simulink model "Foc_model_Matlab_3"  (R2024b)
settings: Solver=FixedStepDiscrete  StartTime=0.0  StopTime=5  FixedStep=Ts_simulink  RelTol=1e-3  EnableMultiTasking=on
PreLoadFcn:
  | mcb_pmsm_foc_hall_S32K144EVB_data;
InitFcn:
  | mbd_s32k_consistency_checks(bdroot(gcs));
model workspace (MAT data in the model file):
  IDC_OVERCURRENT : Simulink.Parameter (value not decoded)
  VDC_OVERVOLTAGE : Simulink.Parameter (value not decoded)
  VDC_UNDERVOLTAGE : Simulink.Parameter (value not decoded)
undefined symbols (not defined in the file or in its folder): Aw, Bw, DiscIntNeverNeededParam, External, inverter, Kcd, Kcq, Kcs, Kid, Kiq, LQFP, mcb_isCodeGenVar, mcb_isSimVar, One, PI_params, pmsm, PU_System, rhow, Shot, sigbuilder_block, TRGMUX_PDB_TRIG, Ts, Ts_motor, Ts_simulink, Ts_speed, tuning
libraries: mbd_s32k1xx_ec_toolbox x39, mcbcontrolslib x9, simulink x6, mcbpositiondecoderlib x6, mbd_msd_ec_toolbox x5, hdlsllib x4, slpidlib x2, mcbhdlpositiondecoderlib x1, mcbplantlib x1, autolibpmsmexterior x1
(part 2 of 3)

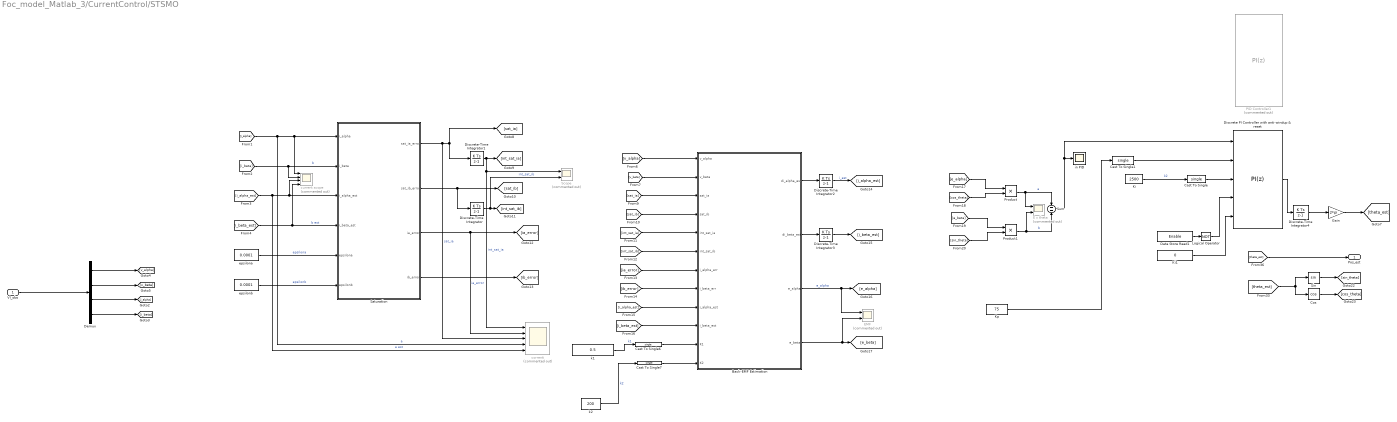
== system Foc_model_Matlab_3/CurrentControl/STSMO ==
  VI_obs : Inport
  Back-EMF Estimation : MATLAB Function  TreatAsAtomicUnit=on
  Cast To Single{,1,6..7} (4 alike) : DataTypeConversion  OutDataTypeStr=single  SaturateOnIntegerOverflow=off  RndMeth=Floor
  Cos : Trigonometry  Operator=cos
  Data Store Read1 : DataStoreRead  DataStoreName=Enable  IndexOptions=Index vector (dialog)  Indices=1  OutputSizes=1
  Demux : Demux
  Discrete PI Controller with anti-windup & reset : slpidlib/PID Controller  Controller=PI  Form=Parallel  TimeDomain=Discrete-time  UseExternalTs=off  SampleTime=-1  IntegratorMethod=Forward Euler  FilterMethod=Forward Euler  ControllerParametersSource=external  P=1  I=1  UseKiTs=off  D=0  UseExternalDerivativeSource=off  N=100  UseFilter=on  TunerSelectOption=Transfer Function Based (PID Tuner App)  InitialConditionSource=external  InitialConditionForIntegrator=0  InitialConditionForFilter=0  DifferentiatorICPrevScaledInput=0  ExternalReset=level  TrackingMode=off  Kt=1  LimitOutput=off  SatLimitsSource=internal  UpperSaturationLimit=1  LowerSaturationLimit=-1  LinearizeAsGain=on  AntiWindupMode=clamping  Kb=1  LimitIntegrator=off  UpperIntegratorSaturationLimit=inf  LowerIntegratorSaturationLimit=-inf  RndMeth=Simplest  POutMin=[]  POutMax=[]  IOutMin=[]  IOutMax=[]  DOutMin=[]  DOutMax=[]  NOutMin=[]  NOutMax=[]  SumOutMin=[]  SumOutMax=[]  SaturationOutDataTypeStr=Inherit: Inherit via back propagation  SaturationOutMin=[]  SaturationOutMax=[]  PParamMin=[]  PParamMax=[]  IParamMin=[]  IParamMax=[]  DParamMin=[]  DParamMax=[]  NParamMin=[]  NParamMax=[]  KbParamMin=[]  KbParamMax=[]  KtParamMin=[]  KtParamMax=[]  KbOutMin=[]  KbOutMax=[]  KtOutMin=[]  KtOutMax=[]  IntegratorOutMin=[]  IntegratorOutMax=[]  FilterOutMin=[]  FilterOutMax=[]  SumI1OutMin=[]  SumI1OutMax=[]  SumI2OutMin=[]  SumI2OutMax=[]  SumI3OutMin=[]  SumI3OutMax=[]  SumI4OutMin=[]  SumI4OutMax=[]  SumDOutMin=[]  SumDOutMax=[]  DifferentiatorOutMin=[]  DifferentiatorOutMax=[]  FilterDiffOutCoefMin=[]  FilterDiffOutCoefMax=[]  ReciprocalOutMin=[]  ReciprocalOutMax=[]  SumDenOutMin=[]  SumDenOutMax=[]  SumNumOutMin=[]  SumNumOutMax=[]  DivideOutMin=[]  DivideOutMax=[]  UdiffTsProdOutMin=[]  UdiffTsProdOutMax=[]  NTsProdOutMin=[]  NTsProdOutMax=[]  UintegralTsProdOutMin=[]  UintegralTsProdOutMax=[]  UngainTsProdOutMin=[]  UngainTsProdOutMax=[]  ClampingZeroOutDataTypeStr=Inherit: Inherit via back propagation  ClampingZeroOutMin=[]  ClampingZeroOutMax=[]  FilterDenConstantOutDataTypeStr=Inherit: Inherit via back propagation  FilterDenConstantOutMin=[]  FilterDenConstantOutMax=[]  PCopyOutDataTypeStr=Inherit: Inherit via back propagation  PCopyOutMin=[]  PCopyOutMax=[]  NCopyOutDataTypeStr=Inherit: Inherit via back propagation  NCopyOutMin=[]  NCopyOutMax=[]  IntegratorContinuousStateAttributes=''  IntegratorStateMustResolveToSignalObject=off  IntegratorRTWStateStorageClass=Auto  FilterContinuousStateAttributes=''  FilterStateMustResolveToSignalObject=off  FilterRTWStateStorageClass=Auto  ParallelPVariant=ExternalParameters  IdealPVariant=Disabled  IVariant=ExternalParameters  DVariant=Disabled  IntegratorVariant=Discrete  SatVariant=Disabled  AWVariant=Passthrough  PCopyVariant=Disabled  TRVariant=Disabled  FdbkBlocksVariant=Forward  IdealPFdbkVariant=Disabled  SatFdbkVariant=Disabled  DerivativeFilterVariant=Disabled  NVariant=Disabled  NCopyVariant=Disabled_SignalSpec  FilterICVariant=Disabled  IntegratorICVariant=ExternalICs  ExternalResetVariant=ExternalReset  TRSumVariant=Passthrough  SumFdbkVariant=Disabled  SumVariant=Sum_PI  TsampFilterVariant=InternalTs  TsampNgainVariant=Passthrough  TsampIntegralVariant=Disabled_SignalSpec  ExternalSaturationOutDataTypeStr=Inherit: Same as second input  DerivativeSourceVariant=Disabled  PreIntVariant=InternalPreInt
  Discrete-Time Integrator{,1..4} (5 alike) : DiscreteIntegrator  SampleTime=-1  ICPrevOutput=DiscIntNeverNeededParam  ICPrevScaledInput=DiscIntNeverNeededParam
  E x theta : Scope  Commented=on  NumInputPorts=2
  EMF : Scope  Commented=on  NumInputPorts=2
  Gain : Gain  Gain=2*pi
  Ki : Constant  Value=2500
  Ki1 : Constant  Value=0  OutDataTypeStr=dataType  SampleTime=-1
  Kp : Constant  Value=75
  Logical Operator : Logic  Operator=NOT  IconShape=distinctive  AllPortsSameDT=off  OutDataTypeStr=boolean
  PID Controller1 : slpidlib/PID Controller  Commented=on  Controller=PI  Form=Parallel  TimeDomain=Discrete-time  UseExternalTs=off  SampleTime=-1  IntegratorMethod=Forward Euler  FilterMethod=Forward Euler  ControllerParametersSource=external  P=1  I=1  UseKiTs=off  D=0  UseExternalDerivativeSource=off  N=100  UseFilter=on  TunerSelectOption=Transfer Function Based (PID Tuner App)  InitialConditionSource=internal  InitialConditionForIntegrator=0  InitialConditionForFilter=0  DifferentiatorICPrevScaledInput=0  ExternalReset=none  TrackingMode=off  Kt=1  LimitOutput=off  SatLimitsSource=internal  UpperSaturationLimit=inf  LowerSaturationLimit=-inf  LinearizeAsGain=on  AntiWindupMode=none  Kb=1  LimitIntegrator=off  UpperIntegratorSaturationLimit=inf  LowerIntegratorSaturationLimit=-inf  POutMin=[]  POutMax=[]  IOutMin=[]  IOutMax=[]  DOutMin=[]  DOutMax=[]  NOutMin=[]  NOutMax=[]  SumOutMin=[]  SumOutMax=[]  SaturationOutMin=[]  SaturationOutMax=[]  PParamMin=[]  PParamMax=[]  IParamMin=[]  IParamMax=[]  DParamMin=[]  DParamMax=[]  NParamMin=[]  NParamMax=[]  KbParamMin=[]  KbParamMax=[]  KtParamMin=[]  KtParamMax=[]  KbOutMin=[]  KbOutMax=[]  KtOutMin=[]  KtOutMax=[]  IntegratorOutMin=[]  IntegratorOutMax=[]  FilterOutMin=[]  FilterOutMax=[]  SumI1OutMin=[]  SumI1OutMax=[]  SumI2OutMin=[]  SumI2OutMax=[]  SumI3OutMin=[]  SumI3OutMax=[]  SumI4OutMin=[]  SumI4OutMax=[]  SumDOutMin=[]  SumDOutMax=[]  DifferentiatorOutMin=[]  DifferentiatorOutMax=[]  FilterDiffOutCoefMin=[]  FilterDiffOutCoefMax=[]  ReciprocalOutMin=[]  ReciprocalOutMax=[]  SumDenOutMin=[]  SumDenOutMax=[]  SumNumOutMin=[]  SumNumOutMax=[]  DivideOutMin=[]  DivideOutMax=[]  UdiffTsProdOutMin=[]  UdiffTsProdOutMax=[]  NTsProdOutMin=[]  NTsProdOutMax=[]  UintegralTsProdOutMin=[]  UintegralTsProdOutMax=[]  UngainTsProdOutMin=[]  UngainTsProdOutMax=[]  ClampingZeroOutDataTypeStr=Inherit: Inherit via back propagation  ClampingZeroOutMin=[]  ClampingZeroOutMax=[]  FilterDenConstantOutDataTypeStr=Inherit: Inherit via back propagation  FilterDenConstantOutMin=[]  FilterDenConstantOutMax=[]  PCopyOutDataTypeStr=Inherit: Inherit via back propagation  PCopyOutMin=[]  PCopyOutMax=[]  NCopyOutDataTypeStr=Inherit: Inherit via back propagation  NCopyOutMin=[]  NCopyOutMax=[]  IntegratorContinuousStateAttributes=''  IntegratorStateMustResolveToSignalObject=off  IntegratorRTWStateStorageClass=Auto  FilterContinuousStateAttributes=''  FilterStateMustResolveToSignalObject=off  FilterRTWStateStorageClass=Auto  ParallelPVariant=ExternalParameters  IdealPVariant=Disabled  IVariant=ExternalParameters  DVariant=Disabled  IntegratorVariant=Discrete  SatVariant=Disabled  AWVariant=Passthrough  PCopyVariant=Disabled  TRVariant=Disabled  FdbkBlocksVariant=Forward  IdealPFdbkVariant=Disabled  SatFdbkVariant=Disabled  DerivativeFilterVariant=Disabled  NVariant=Disabled  NCopyVariant=Disabled_SignalSpec  FilterICVariant=Disabled  IntegratorICVariant=InternalICs  ExternalResetVariant=Disabled  TRSumVariant=Passthrough  SumFdbkVariant=Disabled  SumVariant=Sum_PI  TsampFilterVariant=InternalTs  TsampNgainVariant=Passthrough  TsampIntegralVariant=Disabled_SignalSpec  ExternalSaturationOutDataTypeStr=Inherit: Same as second input  DerivativeSourceVariant=Disabled  PreIntVariant=InternalPreInt
  Product : Product
  Product1 : Product
  "Saturation " : MATLAB Function  TreatAsAtomicUnit=on
  Scope : Scope  Commented=on  NumInputPorts=2
  Sin : Trigonometry
  Sum : Sum  Inputs=--
  correnti : Scope  Commented=on  NumInputPorts=5
  current scope : Scope  Commented=on  NumInputPorts=4
  epsilona : Constant  Value=0.0001
  epsilonb : Constant  Value=0.0001
  in PID : Scope
  k1 : Constant  Value=0.5
  k2 : Constant  Value=200
  Pos_est : Outport
  wires:
  Demux/4 -> [i_beta]
  [i_beta] -> current scope/2, "Saturation "/2(i_beta)  "b"
  "Saturation "/1(sat_ia_error) -> correnti/3, Discrete-Time Integrator1/1, [sat_ia]  "sat_ia"
  "Saturation "/2(sat_ib_error) -> Discrete-Time Integrator/1, [sat_ib]
  "Saturation "/3(ia_error) -> correnti/2, [ia_error]  "ia_error"
  "Saturation "/4(ib_error) -> [ib_error]
  Discrete-Time Integrator/1 -> Scope/2, [int_sat_ib]  "int_sat_ib"
  Back-EMF Estimation/1(di_alpha_est) -> Discrete-Time Integrator2/1
  Back-EMF Estimation/2(di_beta_est) -> Discrete-Time Integrator3/1
  Back-EMF Estimation/3(e_alpha) -> EMF/1, [e_alpha]  "e_alpha"
  Back-EMF Estimation/4(e_beta) -> EMF/2, [e_beta]
  [v_alpha] -> Back-EMF Estimation/1(v_alpha)
  [v_beta] -> Back-EMF Estimation/2(v_beta)
  [sat_ia] -> Back-EMF Estimation/3(sat_ia)
  [sat_ib] -> Back-EMF Estimation/4(sat_ib)
  [int_sat_ia] -> Back-EMF Estimation/5(int_sat_ia)
  [int_sat_ib] -> Back-EMF Estimation/6(int_sat_ib)
  [ia_error] -> Back-EMF Estimation/7(i_alpha_err)
  [ib_error] -> Back-EMF Estimation/8(i_beta_err)
  [sin_theta] -> Product1/2
  [cos_theta] -> Product/2
  VI_obs/1 -> Demux/1
  Sin/1 -> [sin_theta]
  Cos/1 -> [cos_theta]
  [theta_est] -> Pos_est/1
  k1/1 -> Cast To Single6/1  "k1"
  k2/1 -> Cast To Single7/1  "k2"
  epsilona/1 -> "Saturation "/5(epsilona)  "epsilona"
  epsilonb/1 -> "Saturation "/6(epsilonb)  "epsilonb"
  Demux/2 -> [v_beta]
  Demux/1 -> [v_alpha]
  Cast To Single6/1 -> Back-EMF Estimation/11(K1)
  Cast To Single7/1 -> Back-EMF Estimation/12(K2)
  Demux/3 -> [i_alpha]
  [i_alpha_est] -> Back-EMF Estimation/9(i_alpha_est)
  [i_beta_est] -> Back-EMF Estimation/10(i_beta_est)
  Product1/1 -> E x theta/2, Sum/2  "b"
  Discrete-Time Integrator3/1 -> [i_beta_est]
  Discrete-Time Integrator2/1 -> [i_alpha_est]  "i_est"
  [e_beta] -> Product1/1
  [e_alpha] -> Product/1
  [i_beta_est] -> current scope/4, "Saturation "/4(i_beta_est)  "b est"
  [i_alpha_est] -> correnti/5, current scope/3, "Saturation "/3(i_alpha_est)  "a est"
  Kp/1 -> Cast To Single1/1
  [i_alpha] -> correnti/4, current scope/1, "Saturation "/1(i_alpha)  "a"
  Discrete-Time Integrator1/1 -> correnti/1, Scope/1, [int_sat_ia]  "int_sat_ia"
  [theta_est] -> Sin/1, Cos/1
  Product/1 -> E x theta/1, Sum/1  "a"
  Cast To Single1/1 -> Discrete PI Controller with anti-windup & reset/2
  Sum/1 -> Discrete PI Controller with anti-windup & reset/1, in PID/1
  Cast To Single/1 -> Discrete PI Controller with anti-windup & reset/3
  Discrete PI Controller with anti-windup & reset/1 -> Discrete-Time Integrator4/1
  Discrete-Time Integrator4/1 -> Gain/1
  Gain/1 -> [theta_est]
  Ki/1 -> Cast To Single/1  "k2"
  Logical Operator/1 -> Discrete PI Controller with anti-windup & reset/4
  Ki1/1 -> Discrete PI Controller with anti-windup & reset/5
  Data Store Read1/1 -> Logical Operator/1

== system Foc_model_Matlab_3/CurrentControl/Sensor Driver Blocks ==
  Sensor Driver Blocks (codegen) : Subsystem  VariantControl=mcb_isCodeGenVar()
  Sensor Driver Blocks (sim) : Subsystem  VariantControl=mcb_isSimVar()
  Iab_Meas_ADC : Outport

== system Foc_model_Matlab_3/Hall Sensor/CodeGen ==
  Add1 : Sum  Inputs=+++  OutDataTypeStr=Inherit: Inherit via back propagation
  Bit Shift : hdlsllib/Logic and Bit Operations/Bit Shift  mode=Shift Left Logical  N=2
  Bit Shift1 : hdlsllib/Logic and Bit Operations/Bit Shift  mode=Shift Left Logical  N=1
  Data Type Conversion2 : DataTypeConversion  OutDataTypeStr=uint32  SaturateOnIntegerOverflow=off  RndMeth=Floor
  Data Type Conversion3 : DataTypeConversion  OutDataTypeStr=uint32  SaturateOnIntegerOverflow=off  RndMeth=Floor
  Data Type Conversion6 : DataTypeConversion  OutDataTypeStr=uint32  SaturateOnIntegerOverflow=off  RndMeth=Floor
  Digital_Input_HALL_A : mbd_s32k1xx_ec_toolbox/GPIO Blocks/Digital_Input  gpio_pin=PTA1: [PTA1 | Port A I/O]  pull_resistor=None  passive_filter=off
  Digital_Input_HALL_B : mbd_s32k1xx_ec_toolbox/GPIO Blocks/Digital_Input  gpio_pin=PTD10: [PTD10 | Port D I/O]  pull_resistor=None  passive_filter=off
  Digital_Input_HALL_C : mbd_s32k1xx_ec_toolbox/GPIO Blocks/Digital_Input  gpio_pin=PTD11: [PTD11 | Port D I/O]  pull_resistor=None  passive_filter=off
  Out1 : Outport
  wires:
  Bit Shift1/1 -> Add1/2  "HALL_B"
  Digital_Input_HALL_B/1 -> Data Type Conversion2/1
  Add1/1 -> Out1/1
  Data Type Conversion6/1 -> Add1/3  "HALL_C"
  Digital_Input_HALL_A/1 -> Data Type Conversion3/1
  Data Type Conversion2/1 -> Bit Shift1/1
  Bit Shift/1 -> Add1/1  "HALL_A"
  Digital_Input_HALL_C/1 -> Data Type Conversion6/1
  Data Type Conversion3/1 -> Bit Shift/1

== system Foc_model_Matlab_3/Hall Sensor/Sim ==
  Data Type Conversion1 : DataTypeConversion  OutDataTypeStr=uint32  SaturateOnIntegerOverflow=off  RndMeth=Floor
  Ground : Ground
  Out1 : Outport
  wires:
  Ground/1 -> Data Type Conversion1/1
  Data Type Conversion1/1 -> Out1/1

== system Foc_model_Matlab_3/HallCodeGen/Subsystem2 ==
  ADC1_IRQHandler : Subsystem  TreatAsAtomicUnit=on
  ADC1_ISR : mbd_s32k1xx_ec_toolbox/Motor Control Blocks/ADC Blocks/ADC_ISR  instance=1  pri=5  sc1n=C
  Data Store Write : DataStoreWrite  DataStoreName=ADC_A  IndexOptions=Index vector (dialog)  Indices=1  OutputSizes=1
  Data Store Write1 : DataStoreWrite  DataStoreName=ADC_B  IndexOptions=Index vector (dialog)  Indices=1  OutputSizes=1
  Data Type Conversion : DataTypeConversion  OutDataTypeStr=single  SaturateOnIntegerOverflow=off  RndMeth=Floor
  Demux : Demux  Outputs=2
  PDB1_IRQHandler : Subsystem  TreatAsAtomicUnit=on
  PDB1_ISR : mbd_s32k1xx_ec_toolbox/Motor Control Blocks/PDB Blocks/PDB_ISR  Priority=8  pdbModule=0  prioInterrupt=6  regScPdbie=on  regScPdbeie=off  regIdlyIdly=4999
  Terminator{,1..2,6} (4 alike) : Terminator
  FcnCall : Outport  VectorParamsAs1DForOutWhenUnconnected=off
  wires:
  ADC1_IRQHandler/2(ADC_res) -> Data Type Conversion/1
  PDB1_ISR/1 -> PDB1_IRQHandler/Trigger
  PDB1_ISR/3 -> Terminator2/1  "CH0S_ERR"
  PDB1_ISR/4 -> Terminator/1  "CH1S_ERR"
  ADC1_ISR/1 -> ADC1_IRQHandler/Trigger
  PDB1_ISR/2 -> Terminator1/1  "SC_PDBIF"
  ADC1_ISR/2 -> ADC1_IRQHandler/1(ADC_IB)
  ADC1_IRQHandler/1(ADC_Event) -> FcnCall/1
  ADC1_ISR/3 -> Terminator6/1
  Demux/2 -> Data Store Write1/1
  Data Type Conversion/1 -> Demux/1
  Demux/1 -> Data Store Write/1

== system Foc_model_Matlab_3/Hardware Initialization/FAULT ==
  Action Port : ActionPort  ActionPortLabel=else
  LED_GREEN : mbd_s32k1xx_ec_toolbox/GPIO Blocks/Digital_Output  gpio_pin=PTD16: [PTD16 | Port D I/O]  init_val=Low  drive_strength=Low
  LED_RED : mbd_s32k1xx_ec_toolbox/GPIO Blocks/Digital_Output  gpio_pin=PTD15: [PTD15 | Port D I/O]  init_val=Low  drive_strength=Low
  OFF : Constant  OutDataTypeStr=boolean
  ON : Constant  Value=0  OutDataTypeStr=boolean
  wires:
  OFF/1 -> LED_GREEN/1
  ON/1 -> LED_RED/1

== system Foc_model_Matlab_3/Hardware Initialization/GD3000_interrupt ==
  function : TriggerPort  TriggerType=function-call  VariantControl=Variant
  FAULT_write : DataStoreWrite  DataStoreName=FAULT  IndexOptions=Index vector (dialog)  Indices=1  OutputSizes=1
  FTM_PWM_Disable_Enable : mbd_s32k1xx_ec_toolbox/Motor Control Blocks/FTM Blocks/FTM_PWM_Disable_Enable  ftmModule=3  action=Disable
  NOK : Constant  OutDataTypeStr=boolean
  TPP_Functional_Mode : mbd_msd_ec_toolbox/TPP/TPP_Functional_Mode  tppInstance=0  action=Sleep
  wires:
  NOK/1 -> FAULT_write/1

== system Foc_model_Matlab_3/Hardware Initialization/If Action Subsystem ==
  Action Port : ActionPort  ActionPortLabel=if(u1 == 0)
  LED_GREEN : Constant  Value=0  OutDataTypeStr=boolean  SampleTime=-1
  LED_GREEN_ON : mbd_s32k1xx_ec_toolbox/GPIO Blocks/Digital_Output  gpio_pin=PTD16: [PTD16 | Port D I/O]  init_val=Low  drive_strength=Low
  LED_RED : Constant  OutDataTypeStr=boolean  SampleTime=-1
  LED_RED_OFF : mbd_s32k1xx_ec_toolbox/GPIO Blocks/Digital_Output  gpio_pin=PTD15: [PTD15 | Port D I/O]  init_val=Low  drive_strength=Low
  wires:
  LED_GREEN/1 -> LED_GREEN_ON/1
  LED_RED/1 -> LED_RED_OFF/1

== system Foc_model_Matlab_3/Hardware Initialization/enable_FTM_PDB_ADC_triggering ==
  function : TriggerPort  TriggerType=function-call  VariantControl=(inherit)
  Custom code to reload the PDB value : Subsystem  Priority=6  mask(System Outputs){ShowInLibBrowser=0}
      mask prompts: ShowInLibBrowser "Simulink:masks:CustCodeMaskParam1_MP"
      settings: CopyFcn=cccopyfcn(gcb)  OpenFcn=ccopenfcn('System Outputs Function')
      mask Help: eval('feval(''rtwprivate'',''rtwhelpview'',''rtw_sys_outputs_block'')');
      mask Display: disp('System\nOutputs');
  FTM_Init_Trigger_Disable_Enable : mbd_s32k1xx_ec_toolbox/Motor Control Blocks/FTM Blocks/FTM_Init_Trigger_Disable_Enable  Priority=3  ftmModule=3  action=Enable
  FTM_PWM_Disable_Enable : mbd_s32k1xx_ec_toolbox/Motor Control Blocks/FTM Blocks/FTM_PWM_Disable_Enable  Priority=1  ftmModule=3  action=Enable
  PDB0_Enable : mbd_s32k1xx_ec_toolbox/Motor Control Blocks/PDB Blocks/PDB_Enable  Priority=4  pdbModule=0  pdbAction=Enable
  PDB1_Enable : mbd_s32k1xx_ec_toolbox/Motor Control Blocks/PDB Blocks/PDB_Enable  Priority=5  pdbModule=1  pdbAction=Enable
  TPP_ISR_Enable_Disable : mbd_msd_ec_toolbox/TPP/TPP_ISR_Enable_Disable  Priority=7  tppInstance=0  mcuTppIntEn=on  prioInt=15

== system Foc_model_Matlab_3/Inverter and Motor - Plant Model/Codegeneration ==
  Duty_Cycles : Inport
  Ground : Ground
  Ground1 : Ground
  Terminator : Terminator
  Iab_fb_Sim : Outport  VectorParamsAs1DForOutWhenUnconnected=off
  Pos_fb_Sim : Outport  Port=2  VectorParamsAs1DForOutWhenUnconnected=off
  wires:
  Duty_Cycles/1 -> Terminator/1
  Ground/1 -> Iab_fb_Sim/1
  Ground1/1 -> Pos_fb_Sim/1

== system Foc_model_Matlab_3/Inverter and Motor - Plant Model/Simulation ==
  Duty_Cycles : Inport
  Average Inverter : Subsystem
  Load_Profile (Torque) : Subsystem
  RT1 : RateTransition  Deterministic=off  OutPortSampleTime=Ts_simulink
  RT3 : RateTransition  Deterministic=off  OutPortSampleTime=Ts_simulink
  Rate Transition : RateTransition  Deterministic=off  OutPortSampleTime=Ts_motor
  Rate Transition1 : RateTransition  Deterministic=off  OutPortSampleTime=Ts_motor
  Sensor_Measurements : Subsystem
  Surface Mount PMSM : autolibpmsmexterior/Surface Mount PMSM  port_config=Torque  sim_type=Discrete  Ts=Ts_motor  FilePath=surfacepmsm_motordata.m  P=pmsm.p  Rs=pmsm.Rs + inverter.R_board  Ldq_=pmsm.Ld  KConstText=Permanent flux linkage constant (lambda_pm):  lambda_pm=pmsm.FluxPM  Ke=159.9771  Kt=1.323  mechanical=[pmsm.J, pmsm.B, 0]  idq0=[0 0]  theta_init=0  omega_init=0  KConst=pmsm.FluxPM  lambda_pm_calc=pmsm.FluxPM  RefBlkName='autolibpmsmexterior/Surface Mount PMSM'  aMode=5  Ldq="[0.0006      0.0006]"
  Terminator : Terminator
  Iab_fb_Sim : Outport  VectorParamsAs1DForOutWhenUnconnected=off
  Pos_fb_Sim : Outport  Port=2  VectorParamsAs1DForOutWhenUnconnected=off
  wires:
  RT1/1 -> Sensor_Measurements/2(PhaseCurr)
  Surface Mount PMSM/3 -> Terminator/1
  Average Inverter/1(Vabc) -> Rate Transition/1
  Load_Profile (Torque)/1(Load_Trq) -> Rate Transition1/1
  Surface Mount PMSM/2 -> RT1/1  "Iabc"
  RT3/1 -> Sensor_Measurements/1(Info)
  Surface Mount PMSM/1 -> RT3/1
  Rate Transition1/1 -> Surface Mount PMSM/1
  Rate Transition/1 -> Surface Mount PMSM/2
  Duty_Cycles/1 -> Average Inverter/1(Duty_abc)
  Sensor_Measurements/1(Iab_fb) -> Iab_fb_Sim/1
  Sensor_Measurements/2(Pos_fb) -> Pos_fb_Sim/1

== system Foc_model_Matlab_3/Serial Receive/Code Generation ==
  Data Store Read2 : DataStoreRead  DataStoreName=DesiredSpeed  IndexOptions=Index vector (dialog)  Indices=1  OutputSizes=1
  Data Store Read3 : DataStoreRead  DataStoreName=Enable  IndexOptions=Index vector (dialog)  Indices=1  OutputSizes=1
  Data Type Conversion5 : DataTypeConversion  OutDataTypeStr=single  RndMeth=Simplest  SaturateOnIntegerOverflow=off
  Mux1 : Mux  Inputs=2
  rpm2PU : Gain  Gain=1/pmsm.N_max  RndMeth=Simplest
  Data : Outport
  wires:
  Data Store Read3/1 -> Data Type Conversion5/1
  Data Type Conversion5/1 -> Mux1/2
  Mux1/1 -> Data/1
  Data Store Read2/1 -> rpm2PU/1
  rpm2PU/1 -> Mux1/1

== system Foc_model_Matlab_3/Serial Receive/Simulation ==
  Cast To Single1 : DataTypeConversion  OutDataTypeStr=single  SaturateOnIntegerOverflow=off  RndMeth=Floor
  Constant : Constant
  Gain : Gain  Gain=1/pmsm.N_max
  Mux2 : Mux  Inputs=2
  Push Button : PushButtonBlock  ButtonType=Latch  OffValue=0.000000
  Signal Builder : Subsystem  Tag=STV Subsys  LoadFcn=sigbuilder_block('load');  StartFcn=sigbuilder_block('start');  StopFcn=sigbuilder_block('stop');  ClipboardFcn=sigbuilder_block('clipboard');  mask(Sigbuilder block){tuvar=[0:10]}
      mask help: Simulink:masks:SigbuilderBlock_MD
      mask init:
      | if ~strcmp(get_param(bdroot(gcbh),'SimulationStatus'),'stopped') tuvar = sigbuilder_block('maskInit'); end
      settings: CopyFcn=sigbuilder_block('copy');  DeleteFcn=sigbuilder_block('delete');  ModelCloseFcn=sigbuilder_block('modelClose');  PreSaveFcn=sigbuilder_block('preSave');  PauseFcn=sigbuilder_block('pause');  ContinueFcn=sigbuilder_block('continue');  NameChangeFcn=sigbuilder_block('namechange');  OpenFcn=sigbuilder_block('open',[0 0 1152 591.6 ]);  CloseFcn=sigbuilder_block('close');
      mask Display: plot(0, 0, 100, 100,[2, 2, 32, 32, 2], [68, 8, 8, 68, 68],[32, 2], [38, 38], [32, 19, 2],[53, 60, 44], [32, 17, 17, 2],[16, 16, 31, 31]);txt = getActiveGroup(gcbh);text(2, 100, txt,'verticalAlignment', 'top');
  Speed_Ref_Final (rpm)1 : Constant  Value=0.8*pmsm.N_max  OutDataTypeStr=dataType  SampleTime=-1
  Speed_Ref_Init (rpm)1 : Step  Time=0  OutDataTypeStr=single
  Switch : Switch  Criteria=u2 > Threshold  SaturateOnIntegerOverflow=off  InputSameDT=off
  Data : Outport
  wires:
  Mux2/1 -> Data/1
  Speed_Ref_Init (rpm)1/1 -> Mux2/2
  Speed_Ref_Final (rpm)1/1 -> Gain/1
  Switch/1 -> Mux2/1
  Cast To Single1/1 -> Switch/1
  Constant/1 -> Switch/2
  Gain/1 -> Switch/3
  Signal Builder/1(Signal 1) -> Cast To Single1/1

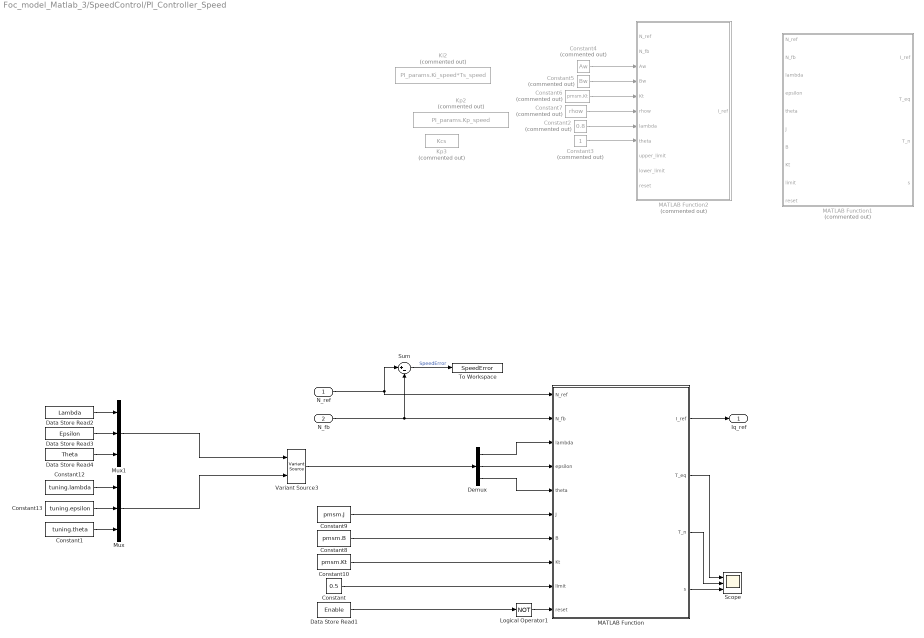
== system Foc_model_Matlab_3/SpeedControl/PI_Controller_Speed ==
  N_ref : Inport
  N_fb : Inport  Port=2
  Constant : Constant  Value=0.5
  Constant1 : Constant  Value=tuning.theta
  Constant10 : Constant  Value=pmsm.Kt
  Constant12 : Constant  Value=tuning.lambda
  Constant13 : Constant  Value=tuning.epsilon
  Constant2 : Constant  Commented=on  Value=0.8
  Constant3 : Constant  Commented=on
  Constant4 : Constant  Commented=on  Value=Aw
  Constant5 : Constant  Commented=on  Value=Bw
  Constant6 : Constant  Commented=on  Value=pmsm.Kt
  Constant7 : Constant  Commented=on  Value=rhow
  Constant8 : Constant  Value=pmsm.B
  Constant9 : Constant  Value=pmsm.J
  Data Store Read2 : DataStoreRead  DataStoreName=Lambda  IndexOptions=Index vector (dialog)  Indices=1  OutputSizes=1
  Data Store Read3 : DataStoreRead  DataStoreName=Epsilon  IndexOptions=Index vector (dialog)  Indices=1  OutputSizes=1
  Data Store Read4 : DataStoreRead  DataStoreName=Theta  IndexOptions=Index vector (dialog)  Indices=1  OutputSizes=1
  Data Store Read1 : DataStoreRead  DataStoreName=Enable  IndexOptions=Index vector (dialog)  Indices=1  OutputSizes=1
  Demux : Demux  Outputs=3
  Ki2 : Constant  Commented=on  Value=PI_params.Ki_speed*Ts_speed  OutDataTypeStr=dataType  SampleTime=-1
  Kp2 : Constant  Commented=on  Value=PI_params.Kp_speed  OutDataTypeStr=dataType  SampleTime=-1
  Kp3 : Constant  Commented=on  Value=Kcs  OutDataTypeStr=dataType  SampleTime=-1
  Logical Operator1 : Logic  Operator=NOT  IconShape=distinctive  AllPortsSameDT=off  OutDataTypeStr=boolean
  MATLAB Function : MATLAB Function  TreatAsAtomicUnit=on
  MATLAB Function1 : MATLAB Function  Commented=on  TreatAsAtomicUnit=on
  MATLAB Function2 : MATLAB Function  Commented=on  TreatAsAtomicUnit=on
  Mux : Mux  Inputs=3
  Mux1 : Mux  Inputs=3
  Scope : Scope  NumInputPorts=3
  Sum : Sum  Inputs=|+-  RndMeth=Simplest  OutDataTypeStr=Inherit: Same as first input
  To Workspace : ToWorkspace  VariableName=SpeedError  SaveFormat=Structure With Time  SampleTime=-1
  Variant Source3 : VariantSource
  Iq_ref : Outport  VectorParamsAs1DForOutWhenUnconnected=off
  wires:
  Sum/1 -> To Workspace/1  "SpeedError"
  Constant/1 -> MATLAB Function/9(limit)
  Logical Operator1/1 -> MATLAB Function/10(reset)
  Constant7/1 -> MATLAB Function2/6(rhow)
  Constant6/1 -> MATLAB Function2/5(Kt)
  Constant5/1 -> MATLAB Function2/4(Bw)
  Constant2/1 -> MATLAB Function2/7(lambda)
  Constant3/1 -> MATLAB Function2/8(theta)
  Constant4/1 -> MATLAB Function2/3(Aw)
  N_ref/1 -> MATLAB Function/1(N_ref), Sum/1
  N_fb/1 -> Sum/2, MATLAB Function/2(N_fb)
  MATLAB Function/1(I_ref) -> Iq_ref/1
  Data Store Read1/1 -> Logical Operator1/1
  Constant8/1 -> MATLAB Function/7(B)
  Constant9/1 -> MATLAB Function/6(J)
  Constant10/1 -> MATLAB Function/8(Kt)
  Data Store Read4/1 -> Mux1/3
  MATLAB Function/2(T_eq) -> Scope/1
  MATLAB Function/3(T_n) -> Scope/2
  MATLAB Function/4(s) -> Scope/3
  Constant12/1 -> Mux/1
  Constant13/1 -> Mux/2
  Constant1/1 -> Mux/3
  Demux/2 -> MATLAB Function/4(epsilon)
  Mux/1 -> Variant Source3/2
  Mux1/1 -> Variant Source3/1
  Data Store Read2/1 -> Mux1/1
  Data Store Read3/1 -> Mux1/2
  Variant Source3/1 -> Demux/1
  Demux/1 -> MATLAB Function/3(lambda)
  Demux/3 -> MATLAB Function/5(theta)

== system Foc_model_Matlab_3/SpeedControl/Speed_Ref_Selector ==
  Speed_Ref_In : Inport
  Speed_Ref_Open : Inport  Port=2
  Data Store Read1 : DataStoreRead  DataStoreName=Enable  IndexOptions=Index vector (dialog)  Indices=1  OutputSizes=1
  Data Type Conversion : DataTypeConversion  OutDataTypeStr=single  SaturateOnIntegerOverflow=off  RndMeth=Floor
  IIR Filter : mcbcontrolslib/IIR Filter  Commented=through  VariantControl=Low Pass Filter  VariantSelect=Low-pass  FilterConstantInputType=Specify via dialog  Filter_constant=0.01  advancedSettings=off  Ts=50e-6  cutOff_freq=32.1525
  Switch : Switch  Criteria=u2 > Threshold  Threshold=0.5  SaturateOnIntegerOverflow=off  InputSameDT=off
  Speed_Ref_PU : Outport
  wires:
  IIR Filter/1 -> Speed_Ref_PU/1
  Speed_Ref_Open/1 -> Switch/3
  Speed_Ref_In/1 -> Switch/1
  Data Type Conversion/1 -> Switch/2
  Data Store Read1/1 -> Data Type Conversion/1
  Switch/1 -> IIR Filter/1

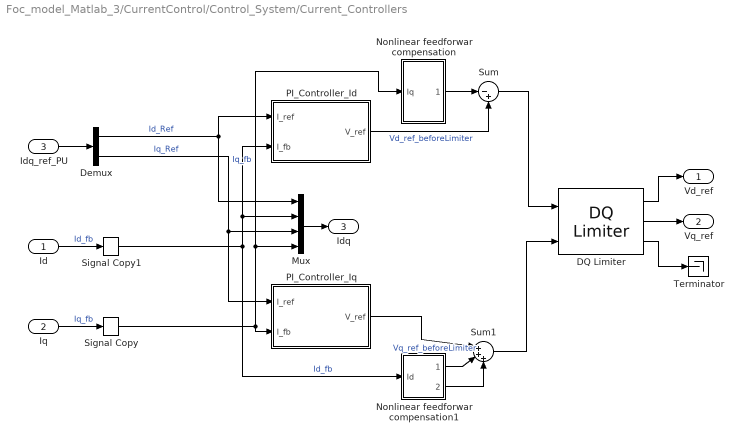
== system Foc_model_Matlab_3/CurrentControl/Control_System/Current_Controllers ==
  Id : Inport
  Iq : Inport  Port=2
  Idq_ref_PU : Inport  Port=3
  DQ Limiter : mcbcontrolslib/DQ Limiter  satMethodInputType=Specify via dialog  satMethodSelected=D-Q equivalence  satLimitInputType=Specify via dialog  Vmax=0.95
  Demux : Demux  Outputs=2
  Mux : Mux
  Nonlinear feedforwar compensation : Subsystem
  Nonlinear feedforwar compensation1 : Subsystem
  PI_Controller_Id : Subsystem
  PI_Controller_Iq : Subsystem
  Signal Copy : SignalConversion  OverrideOpt=off
  Signal Copy1 : SignalConversion  OverrideOpt=off
  Sum : Sum  Inputs=|-+
  Sum1 : Sum  Inputs=|+++
  Terminator : Terminator
  Vd_ref : Outport  VectorParamsAs1DForOutWhenUnconnected=off
  Vq_ref : Outport  Port=2  VectorParamsAs1DForOutWhenUnconnected=off
  Idq : Outport  Port=3  VectorParamsAs1DForOutWhenUnconnected=off
  wires:
  Idq_ref_PU/1 -> Demux/1
  DQ Limiter/2 -> Vq_ref/1
  DQ Limiter/1 -> Vd_ref/1
  DQ Limiter/3 -> Terminator/1
  Id/1 -> Signal Copy1/1  "Id_fb"
  Iq/1 -> Signal Copy/1  "Iq_fb"
  Mux/1 -> Idq/1
  Nonlinear feedforwar compensation/1(Out1) -> Sum/1
  PI_Controller_Id/1(V_ref) -> Sum/2  "Vd_ref_beforeLimiter"
  Sum/1 -> DQ Limiter/1
  Nonlinear feedforwar compensation1/2(Out2) -> Sum1/3
  Nonlinear feedforwar compensation1/1(Out1) -> Sum1/2
  PI_Controller_Iq/1(V_ref) -> Sum1/1  "Vq_ref_beforeLimiter"
  Sum1/1 -> DQ Limiter/2
  Signal Copy/1 -> Nonlinear feedforwar compensation/1(Iq), Mux/4, PI_Controller_Iq/2(I_fb)  "Iq_fb"
  Signal Copy1/1 -> Nonlinear feedforwar compensation1/1(Id), PI_Controller_Id/2(I_fb), Mux/2  "Id_fb"
  Demux/1 -> PI_Controller_Id/1(I_ref), Mux/1  "Id_Ref"
  Demux/2 -> PI_Controller_Iq/1(I_ref), Mux/3  "Iq_Ref"

== system Foc_model_Matlab_3/CurrentControl/Input Scaling/Read_Sensor (codegen) ==
  Iab_meas_ADC : Inport
  Iab_Sim : Inport  Port=2
  Pos_Sim : Inport  Port=3
  Calculate Position from Hall : Subsystem
  Convert ADC value to PU : Subsystem
  Terminator : Terminator
  Terminator1 : Terminator
  Iab_Meas_PU : Outport  VectorParamsAs1DForOutWhenUnconnected=off
  Pos_PU : Outport  Port=2  VectorParamsAs1DForOutWhenUnconnected=off
  Speed_PU : Outport  Port=3  VectorParamsAs1DForOutWhenUnconnected=off
  wires:
  Iab_Sim/1 -> Terminator/1
  Calculate Position from Hall/1(Pos_PU) -> Pos_PU/1
  Iab_meas_ADC/1 -> Convert ADC value to PU/1(Iab_meas_ADC)
  Convert ADC value to PU/1(Iab_meas_PU) -> Iab_Meas_PU/1
  Pos_Sim/1 -> Terminator1/1
  Calculate Position from Hall/2(Speed_PU) -> Speed_PU/1

== system Foc_model_Matlab_3/CurrentControl/Input Scaling/Read_Sensor (sim) ==
  Iab_meas_ADC : Inport  OutDataTypeStr=uint16
  Iab_Sim : Inport  Port=2
  Pos_Sim : Inport  Port=3
  Convert ADC value to PU : Subsystem
  Subsystem : Subsystem
  Terminator : Terminator
  Iab_Meas_PU : Outport  VectorParamsAs1DForOutWhenUnconnected=off
  Pos_PU : Outport  Port=2  VectorParamsAs1DForOutWhenUnconnected=off
  Speed_PU : Outport  Port=3  VectorParamsAs1DForOutWhenUnconnected=off
  wires:
  Iab_meas_ADC/1 -> Terminator/1
  Pos_Sim/1 -> Subsystem/1(Pos_Sim)
  Subsystem/1(Theta) -> Pos_PU/1
  Subsystem/2(Speed) -> Speed_PU/1
  Convert ADC value to PU/1(Iab_meas_PU) -> Iab_Meas_PU/1
  Iab_Sim/1 -> Convert ADC value to PU/1(Iab_meas_ADC)

== system Foc_model_Matlab_3/CurrentControl/Sensor Driver Blocks/Sensor Driver Blocks (codegen) ==
  Data Store Read : DataStoreRead  DataStoreName=ADC_A  IndexOptions=Index vector (dialog)  Indices=1  OutputSizes=1
  Data Store Read1 : DataStoreRead  DataStoreName=ADC_B  IndexOptions=Index vector (dialog)  Indices=1  OutputSizes=1
  Mux1 : Mux  Inputs=2
  Iab_Meas_ADC : Outport
  wires:
  Mux1/1 -> Iab_Meas_ADC/1
  Data Store Read/1 -> Mux1/1
  Data Store Read1/1 -> Mux1/2

== system Foc_model_Matlab_3/CurrentControl/Sensor Driver Blocks/Sensor Driver Blocks (sim) ==
  Ground : Ground
  Iab_Meas_ADC : Outport
  wires:
  Ground/1 -> Iab_Meas_ADC/1

== system Foc_model_Matlab_3/HallCodeGen/Subsystem2/ADC1_IRQHandler ==
  ADC_IB : Inport
  function : TriggerPort  TriggerType=function-call  VariantControl=(inherit)
  ADC_AD4_IA : mbd_s32k1xx_ec_toolbox/Motor Control Blocks/ADC Blocks/ADC_Start  Priority=2  instance=0  adc_r=A  adc_chan=PTB0: [ADC0_SE4 | ADC Single Ended Input]  aien=off  mcuTargetUpdate=on
  ADC_AD6_IDC : mbd_s32k1xx_ec_toolbox/Motor Control Blocks/ADC Blocks/ADC_Start  Priority=4  instance=1  adc_r=B  adc_chan=PTD4: [ADC1_SE6 | ADC Single Ended Input]  aien=off  mcuTargetUpdate=on
  ADC_AD7_VDC : mbd_s32k1xx_ec_toolbox/Motor Control Blocks/ADC Blocks/ADC_Start  Priority=3  instance=1  adc_r=A  adc_chan=PTB12: [ADC1_SE7 | ADC Single Ended Input]  aien=off  mcuTargetUpdate=on
  ADC_IRQHandlerProfiler : mbd_s32k1xx_ec_toolbox/Utility Blocks/Profiler_Function  profile_indx=2
  FTM_Init_Trigger_Disable : mbd_s32k1xx_ec_toolbox/Motor Control Blocks/FTM Blocks/FTM_Init_Trigger_Disable_Enable  Priority=1  ftmModule=3  action=Disable
  FaultDetection : Subsystem  TreatAsAtomicUnit=on
  Function-Call Generator : simulink/Ports & Subsystems/Function-Call Generator  sample_time=-1  numberOfIterations=1  DisallowWideOutput=off
  Mux1 : Mux  Inputs=2
  ADC_Event : Outport  VectorParamsAs1DForOutWhenUnconnected=off
  ADC_res : Outport  Port=2  VectorParamsAs1DForOutWhenUnconnected=off
  wires:
  ADC_AD4_IA/1 -> Mux1/1  "ADC_IA"
  ADC_AD7_VDC/1 -> FaultDetection/1(Vdc)  "ADC_VDC"
  ADC_AD6_IDC/1 -> FaultDetection/2(Idc)  "ADC_IDC"
  Function-Call Generator/1 -> ADC_Event/1
  ADC_IB/1 -> Mux1/2  "ADC_IB"
  Mux1/1 -> ADC_res/1

== system Foc_model_Matlab_3/HallCodeGen/Subsystem2/PDB1_IRQHandler ==
  function : TriggerPort  TriggerType=function-call  VariantControl=(inherit)
  FTM_Init_Trigger_Enable : mbd_s32k1xx_ec_toolbox/Motor Control Blocks/FTM Blocks/FTM_Init_Trigger_Disable_Enable  ftmModule=3  action=Enable

== system Foc_model_Matlab_3/Hardware Initialization/enable_FTM_PDB_ADC_triggering/Custom code to reload the PDB value ==

== system Foc_model_Matlab_3/Inverter and Motor - Plant Model/Simulation/Average Inverter ==
  Duty_abc : Inport
  Average-Value Inverter : mcbplantlib/Average-Value Inverter
  Constant2 : Constant  Value=inverter.V_dc  OutDataTypeStr=single  SampleTime=-1
  Data Type Conversion1 : DataTypeConversion  OutDataTypeStr=single  RndMeth=Simplest  SaturateOnIntegerOverflow=off
  Rate Transition3 : RateTransition  Deterministic=off  OutPortSampleTime=Ts_inverter
  Vabc : Outport  VectorParamsAs1DForOutWhenUnconnected=off
  wires:
  Data Type Conversion1/1 -> Rate Transition3/1
  Duty_abc/1 -> Data Type Conversion1/1
  Rate Transition3/1 -> Average-Value Inverter/1
  Constant2/1 -> Average-Value Inverter/2
  Average-Value Inverter/1 -> Vabc/1

== system Foc_model_Matlab_3/Inverter and Motor - Plant Model/Simulation/Load_Profile (Torque) ==
  Constant : Constant  Value=0.05*pmsm.T_rated
  Data Type Conversion : DataTypeConversion  OutDataTypeStr=single  SaturateOnIntegerOverflow=off  RndMeth=Floor
  IIR Filter : mcbcontrolslib/IIR Filter  Commented=through  VariantControl=Low Pass Filter  VariantSelect=Low-pass  FilterConstantInputType=Specify via dialog  Filter_constant=0.01  advancedSettings=off  Ts=50e-6  cutOff_freq=32.1525
  T_load : Step  Commented=on  Time=0  Before=0.05*pmsm.T_rated  After=0.5*pmsm.T_rated  SampleTime=Ts_simulink
  Load_Trq : Outport  VectorParamsAs1DForOutWhenUnconnected=off
  wires:
  Data Type Conversion/1 -> IIR Filter/1
  IIR Filter/1 -> Load_Trq/1
  Constant/1 -> Data Type Conversion/1

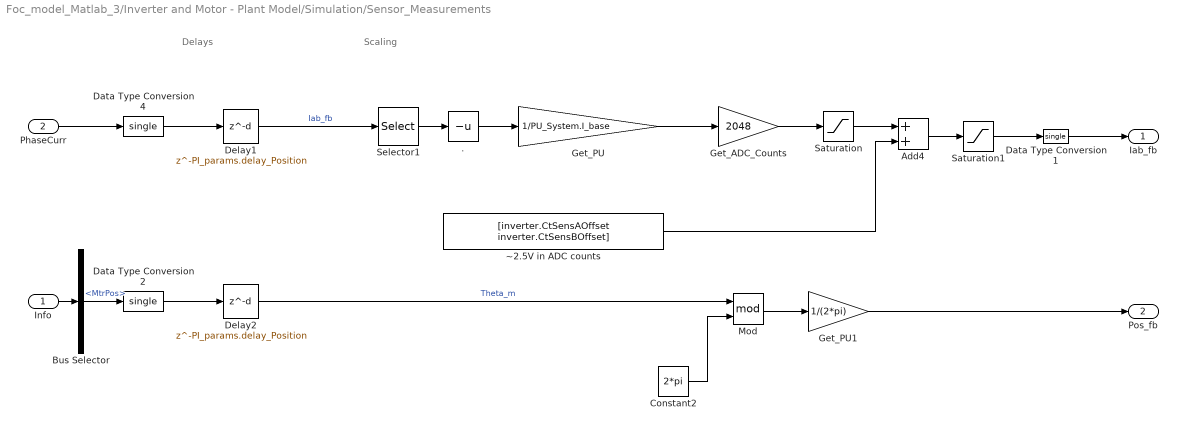
== system Foc_model_Matlab_3/Inverter and Motor - Plant Model/Simulation/Sensor_Measurements ==
  note: Scaling
  note: Delays
  Info : Inport
  PhaseCurr : Inport  Port=2
  . : UnaryMinus
  Add4 : Sum  OutDataTypeStr=uint16
  Bus Selector : BusSelector  OutputSignals=MtrPos
  Constant2 : Constant  Value=2*pi  OutDataTypeStr=single  SampleTime=-1
  Data Type Conversion1 : DataTypeConversion  OutDataTypeStr=single  SaturateOnIntegerOverflow=off  RndMeth=Floor
  Data Type Conversion2 : DataTypeConversion  OutDataTypeStr=single  RndMeth=Simplest  SaturateOnIntegerOverflow=off
  Data Type Conversion4 : DataTypeConversion  OutDataTypeStr=single  RndMeth=Simplest  SaturateOnIntegerOverflow=off
  Delay1 : Delay  DelayLength=PI_params.delay_Position
  Delay2 : Delay  DelayLength=PI_params.delay_Position
  Get_ADC_Counts : Gain  Gain=2048  RndMeth=Simplest  OutDataTypeStr=Inherit: Same as input
  Get_PU : Gain  Gain=1/PU_System.I_base  RndMeth=Simplest
  Get_PU1 : Gain  Gain=1/(2*pi)  OutDataTypeStr=dataType  RndMeth=Simplest
  Mod : Math  Operator=mod
  Saturation : Saturate  UpperLimit=2048  LowerLimit=-2048
  Saturation1 : Saturate  UpperLimit=4095  LowerLimit=0
  Selector1 : Selector  InputPortWidth=3  IndexOptions=Index vector (dialog)  Indices=[1 2]  OutputSizes=1
  ~2.5V in ADC counts : Constant  Value=[inverter.CtSensAOffset inverter.CtSensBOffset]  OutDataTypeStr=uint16  SampleTime=-1
  Iab_fb : Outport  VectorParamsAs1DForOutWhenUnconnected=off
  Pos_fb : Outport  Port=2  VectorParamsAs1DForOutWhenUnconnected=off
  wires:
  Get_ADC_Counts/1 -> Saturation/1
  Saturation1/1 -> Data Type Conversion1/1
  Add4/1 -> Saturation1/1
  ~2.5V in ADC counts/1 -> Add4/2
  Delay1/1 -> Selector1/1  "Iab_fb"
  Saturation/1 -> Add4/1
  Data Type Conversion4/1 -> Delay1/1
  PhaseCurr/1 -> Data Type Conversion4/1
  Get_PU/1 -> Get_ADC_Counts/1
  Info/1 -> Bus Selector/1
  Bus Selector/1 -> Data Type Conversion2/1  "<MtrPos>"
  Data Type Conversion2/1 -> Delay2/1
  Delay2/1 -> Mod/1  "Theta_m"
  Get_PU1/1 -> Pos_fb/1
  ./1 -> Get_PU/1
  Mod/1 -> Get_PU1/1
  Constant2/1 -> Mod/2
  Data Type Conversion1/1 -> Iab_fb/1
  Selector1/1 -> ./1

== system Foc_model_Matlab_3/Serial Receive/Simulation/Signal Builder ==
  Demux : Demux  Tag=STV Demux  Outputs=1
      settings: DisplayOption=none
  FromWs : FromWorkspace  Tag=STV FromWs  VariableName=tuvar  SampleTime=-1  OutputAfterFinalValue=Setting to zero
      SigBuilderData=|
      | common.afterFinalStr = 'Set to zero'
      | common.sampleTime = '-1'
      | dataSet.timeRange = [0 10]
      | dataSet.name = 'Group 1'
      | sbobj.Groups.Name = 'Group 1'
      | sbobj.Groups.Signals.Name = 'Signal 1'
      | sbobj.Groups.Signals.XData = [0 0.5 2 6 10]
      | sbobj.Groups.Signals.YData = [0 0 0.8 0.8 0.805]
  Signal 1 : Outport  Tag=STV Outport
  wires:
  Demux/1 -> Signal 1/1
  FromWs/1 -> Demux/1

== system Foc_model_Matlab_3/CurrentControl/Control_System/Current_Controllers/Nonlinear feedforwar compensation ==
  Iq : Inport
  Gain : Gain  Gain=pmsm.Lq
  Gain1 : Gain  Gain=pmsm.p
  Product : Product
  Out1 : Outport
  wires:
  Gain1/1 -> Product/1
  Product/1 -> Gain/1
  Iq/1 -> Product/2
  [Speed_fb] -> Gain1/1
  Gain/1 -> Out1/1

== system Foc_model_Matlab_3/CurrentControl/Control_System/Current_Controllers/Nonlinear feedforwar compensation1 ==
  Id : Inport
  Cast To Single : DataTypeConversion  OutDataTypeStr=single  SaturateOnIntegerOverflow=off  RndMeth=Floor
  Constant4 : Constant  Value=pmsm.FluxPM
  Gain : Gain  Gain=pmsm.Ld
  Gain1 : Gain  Gain=pmsm.p
  Product : Product
  Product1 : Product
  Out1 : Outport
  Out2 : Outport  Port=2
  wires:
  Gain1/1 -> Product1/2, Product/1
  Id/1 -> Product/2
  [Speed_fb] -> Gain1/1
  Constant4/1 -> Product1/1
  Product/1 -> Gain/1
  Product1/1 -> Cast To Single/1
  Cast To Single/1 -> Out1/1
  Gain/1 -> Out2/1

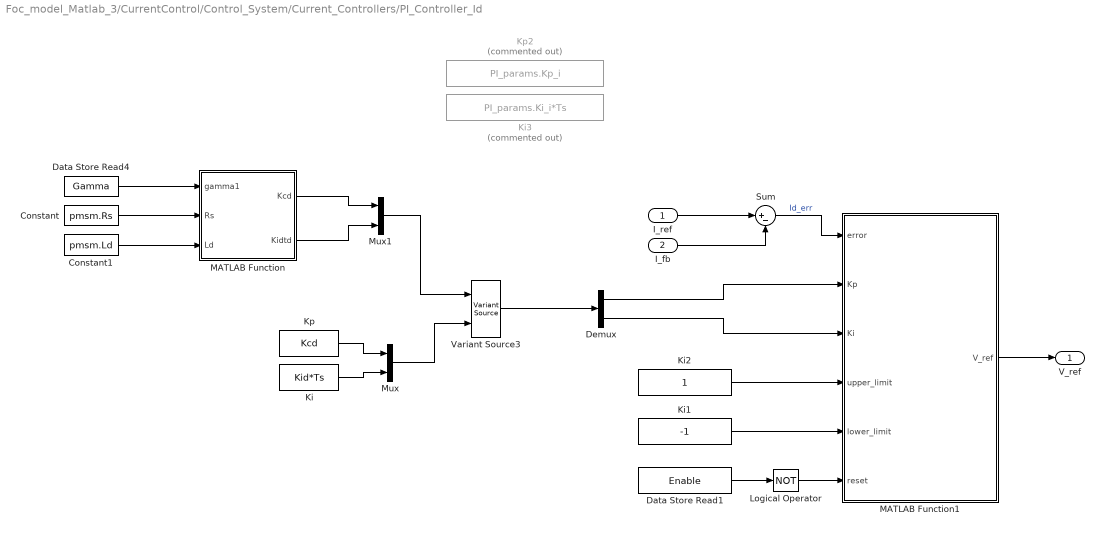
== system Foc_model_Matlab_3/CurrentControl/Control_System/Current_Controllers/PI_Controller_Id ==
  I_ref : Inport
  I_fb : Inport  Port=2
  Constant : Constant  Value=pmsm.Rs
  Constant1 : Constant  Value=pmsm.Ld
  Data Store Read4 : DataStoreRead  DataStoreName=Gamma  IndexOptions=Index vector (dialog)  Indices=1  OutputSizes=1
  Data Store Read1 : DataStoreRead  DataStoreName=Enable  IndexOptions=Index vector (dialog)  Indices=1  OutputSizes=1
  Demux : Demux  Outputs=2
  Ki : Constant  Value=Kid*Ts  OutDataTypeStr=dataType  SampleTime=-1
  Ki1 : Constant  Value=-1  OutDataTypeStr=dataType  SampleTime=-1
  Ki2 : Constant  OutDataTypeStr=dataType  SampleTime=-1
  Ki3 : Constant  Commented=on  Value=PI_params.Ki_i*Ts  OutDataTypeStr=dataType  SampleTime=-1
  Kp : Constant  Value=Kcd  OutDataTypeStr=dataType  SampleTime=-1
  Kp2 : Constant  Commented=on  Value=PI_params.Kp_i  OutDataTypeStr=dataType  SampleTime=-1
  Logical Operator : Logic  Operator=NOT  IconShape=distinctive  AllPortsSameDT=off  OutDataTypeStr=boolean
  MATLAB Function : MATLAB Function  TreatAsAtomicUnit=on
  MATLAB Function1 : MATLAB Function  TreatAsAtomicUnit=on
  Mux : Mux  Inputs=2
  Mux1 : Mux  Inputs=2
  Sum : Sum  Inputs=|+-  OutDataTypeStr=Inherit: Same as first input
  Variant Source3 : VariantSource
  V_ref : Outport  VectorParamsAs1DForOutWhenUnconnected=off
  wires:
  MATLAB Function1/1(V_ref) -> V_ref/1
  I_ref/1 -> Sum/1
  Ki1/1 -> MATLAB Function1/5(lower_limit)
  Sum/1 -> MATLAB Function1/1(error)  "Id_err"
  Data Store Read1/1 -> Logical Operator/1
  I_fb/1 -> Sum/2
  Logical Operator/1 -> MATLAB Function1/6(reset)
  Ki2/1 -> MATLAB Function1/4(upper_limit)
  Demux/2 -> MATLAB Function1/3(Ki)
  Demux/1 -> MATLAB Function1/2(Kp)
  Variant Source3/1 -> Demux/1
  Kp/1 -> Mux/1
  Ki/1 -> Mux/2
  Mux/1 -> Variant Source3/2
  Mux1/1 -> Variant Source3/1
  MATLAB Function/2(Kidtd) -> Mux1/2
  MATLAB Function/1(Kcd) -> Mux1/1
  Data Store Read4/1 -> MATLAB Function/1(gamma1)
  Constant/1 -> MATLAB Function/2(Rs)
  Constant1/1 -> MATLAB Function/3(Ld)

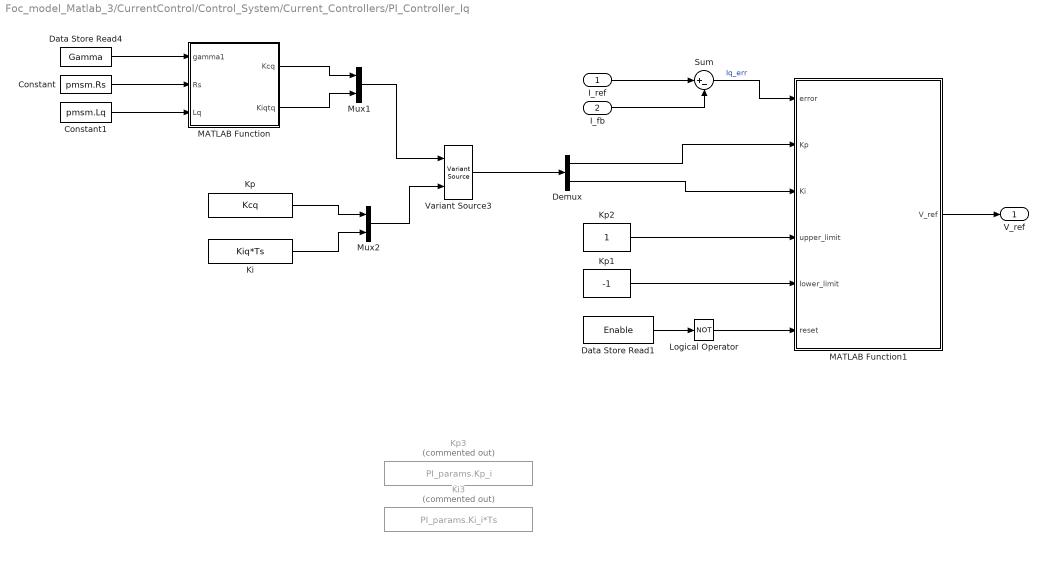
== system Foc_model_Matlab_3/CurrentControl/Control_System/Current_Controllers/PI_Controller_Iq ==
  I_ref : Inport
  I_fb : Inport  Port=2
  Constant : Constant  Value=pmsm.Rs
  Constant1 : Constant  Value=pmsm.Lq
  Data Store Read4 : DataStoreRead  DataStoreName=Gamma  IndexOptions=Index vector (dialog)  Indices=1  OutputSizes=1
  Data Store Read1 : DataStoreRead  DataStoreName=Enable  IndexOptions=Index vector (dialog)  Indices=1  OutputSizes=1
  Demux : Demux  Outputs=2
  Ki : Constant  Value=Kiq*Ts  OutDataTypeStr=dataType  SampleTime=-1
  Ki3 : Constant  Commented=on  Value=PI_params.Ki_i*Ts  OutDataTypeStr=dataType  SampleTime=-1
  Kp : Constant  Value=Kcq  OutDataTypeStr=dataType  SampleTime=-1
  Kp1 : Constant  Value=-1  OutDataTypeStr=dataType  SampleTime=-1
  Kp2 : Constant  OutDataTypeStr=dataType  SampleTime=-1
  Kp3 : Constant  Commented=on  Value=PI_params.Kp_i  OutDataTypeStr=dataType  SampleTime=-1
  Logical Operator : Logic  Operator=NOT  IconShape=distinctive  AllPortsSameDT=off  OutDataTypeStr=boolean
  MATLAB Function : MATLAB Function  TreatAsAtomicUnit=on
  MATLAB Function1 : MATLAB Function  TreatAsAtomicUnit=on
  Mux1 : Mux  Inputs=2
  Mux2 : Mux  Inputs=2
  Sum : Sum  Inputs=|+-  OutDataTypeStr=Inherit: Same as first input
  Variant Source3 : VariantSource
  V_ref : Outport  VectorParamsAs1DForOutWhenUnconnected=off
  wires:
  MATLAB Function1/1(V_ref) -> V_ref/1
  Kp1/1 -> MATLAB Function1/5(lower_limit)
  Data Store Read1/1 -> Logical Operator/1
  Sum/1 -> MATLAB Function1/1(error)  "Iq_err"
  Logical Operator/1 -> MATLAB Function1/6(reset)
  I_fb/1 -> Sum/2
  I_ref/1 -> Sum/1
  Kp2/1 -> MATLAB Function1/4(upper_limit)
  Constant1/1 -> MATLAB Function/3(Lq)
  MATLAB Function/1(Kcq) -> Mux1/1
  Data Store Read4/1 -> MATLAB Function/1(gamma1)
  Demux/1 -> MATLAB Function1/2(Kp)
  Mux2/1 -> Variant Source3/2
  Demux/2 -> MATLAB Function1/3(Ki)
  Mux1/1 -> Variant Source3/1
  Constant/1 -> MATLAB Function/2(Rs)
  MATLAB Function/2(Kiqtq) -> Mux1/2
  Variant Source3/1 -> Demux/1
  Ki/1 -> Mux2/2
  Kp/1 -> Mux2/1

== system Foc_model_Matlab_3/CurrentControl/Input Scaling/Read_Sensor (codegen)/Calculate Position from Hall ==
  Atomic Hall Reading : Subsystem  TreatAsAtomicUnit=on
  Data Store Write2 : DataStoreWrite  Priority=2  DataStoreName=HallStateChangeFlag  IndexOptions=Index vector (dialog)  Indices=1  OutputSizes=1
  Hall Speed and Position : mcbpositiondecoderlib/Hall Speed and Position  blkExecutionType=Speed and position  CounterSize=16 bits  ClkFreq=80000000/128  BlkSampleTime=Ts  PolePairs=pmsm.p  MinSpeed=100  HallInterruptConfig=Every 60 Degrees  SpeedUnit=Per unit  PerUnitSpeed=pmsm.N_max  SpeedDataType=dataType  hallSequence=CBA  Sequence=[6,4,5,1,3,2]  EnableSecondOrder=1st Order  PositionUnit=Per unit  PositionDataType=dataType
  Mechanical to Electrical Position : mcbpositiondecoderlib/Mechanical to Electrical Position  PolePairsInputType=Specify via dialog  NrPP=1  selectedRange=Per unit  MechOfstInputType=Specify via dialog  mechOffsetIn=pmsm.PositionOffset  maxAngleIn=1  InputDataType=dataType  VariantSelect=floating-point
  Pos_PU : Outport  InitialOutput=0  VectorParamsAs1DForOutWhenUnconnected=off
  Speed_PU : Outport  Port=2  InitialOutput=0  VectorParamsAs1DForOutWhenUnconnected=off
  wires:
  Hall Speed and Position/3 -> Data Store Write2/1
  Hall Speed and Position/1 -> Mechanical to Electrical Position/1  "ThetaHalls"
  Mechanical to Electrical Position/1 -> Pos_PU/1
  Atomic Hall Reading/1(HallState) -> Hall Speed and Position/1  "HallVal"
  Atomic Hall Reading/2(Count) -> Hall Speed and Position/2  "CntHallDecoder"
  Atomic Hall Reading/3(SpeedCount) -> Hall Speed and Position/3
  Atomic Hall Reading/4(Dir) -> Hall Speed and Position/4
  Atomic Hall Reading/5(SpeedValidity) -> Hall Speed and Position/5
  Atomic Hall Reading/6(Hallchange) -> Hall Speed and Position/6
  Hall Speed and Position/2 -> Speed_PU/1  "SpeedMeasured"

== system Foc_model_Matlab_3/CurrentControl/Input Scaling/Read_Sensor (codegen)/Convert ADC value to PU ==
  Iab_meas_ADC : Inport
  Add : Sum  Inputs=+-
  Data Store Read : DataStoreRead  DataStoreName=IaOffset  IndexOptions=Index vector (dialog)  Indices=1  OutputSizes=1
  Data Store Read1 : DataStoreRead  DataStoreName=IbOffset  IndexOptions=Index vector (dialog)  Indices=1  OutputSizes=1
  Data Type Conversion2 : DataTypeConversion  OutDataTypeStr=single  SaturateOnIntegerOverflow=off  RndMeth=Floor
  Multiply : Gain  Gain=1/2048
  Mux : Mux  Inputs=2
  Iab_meas_PU : Outport  InitialOutput=0  VectorParamsAs1DForOutWhenUnconnected=off
  wires:
  Data Store Read1/1 -> Mux/2
  Data Store Read/1 -> Mux/1
  Add/1 -> Multiply/1  "I_ab_afterOffset"
  Iab_meas_ADC/1 -> Data Type Conversion2/1
  Mux/1 -> Add/1
  Data Type Conversion2/1 -> Add/2
  Multiply/1 -> Iab_meas_PU/1

== system Foc_model_Matlab_3/CurrentControl/Input Scaling/Read_Sensor (sim)/Convert ADC value to PU ==
  Iab_meas_ADC : Inport
  Add : Sum  Inputs=+-  OutDataTypeStr=single
  Data Store Read : DataStoreRead  DataStoreName=IaOffset  IndexOptions=Index vector (dialog)  Indices=1  OutputSizes=1
  Data Store Read1 : DataStoreRead  DataStoreName=IbOffset  IndexOptions=Index vector (dialog)  Indices=1  OutputSizes=1
  Data Type Conversion1 : DataTypeConversion  OutDataTypeStr=single  SaturateOnIntegerOverflow=off  RndMeth=Floor
  Multiply : Gain  Gain=1/2048  OutDataTypeStr=single
  Mux : Mux  Inputs=2
  Iab_meas_PU : Outport  InitialOutput=0  VectorParamsAs1DForOutWhenUnconnected=off
  wires:
  Data Store Read1/1 -> Mux/2
  Data Store Read/1 -> Mux/1
  Iab_meas_ADC/1 -> Data Type Conversion1/1
  Mux/1 -> Add/1
  Add/1 -> Multiply/1
  Multiply/1 -> Iab_meas_PU/1
  Data Type Conversion1/1 -> Add/2

== system Foc_model_Matlab_3/CurrentControl/Input Scaling/Read_Sensor (sim)/Subsystem ==
  Pos_Sim : Inport
  IIR Filter : mcbcontrolslib/IIR Filter  Commented=through  VariantControl=Low Pass Filter  VariantSelect=Low-pass  FilterConstantInputType=Specify via dialog  Filter_constant=0.01  advancedSettings=off  Ts=50e-6  cutOff_freq=32.1525
  Mechanical to Electrical Position : mcbpositiondecoderlib/Mechanical to Electrical Position  PolePairsInputType=Specify via dialog  NrPP=pmsm.p  selectedRange=Per unit  MechOfstInputType=Specify via dialog  mechOffsetIn=0  maxAngleIn=1  InputDataType=dataType  VariantSelect=floating-point
  Speed Measurement : mcbpositiondecoderlib/Speed Measurement  PositionUnit=Per unit  PositionScalingDatatype=uint32  SpeedCalculationMode=Time interval for speed calculation  SampleTimeAsync=Ts  MaximumApplicationSpeed=6000  SpeedResolution=5e-6  DelayLength=10  MaximumMeasurableSpeed=29999  MeasurableSpeedResolution=1.397e-05  SpeedUnit=Per unit based on dialog  PerUnitSpeed=pmsm.N_max  SpeedDataType=single
  Theta : Outport
  Speed : Outport  Port=2
  wires:
  Mechanical to Electrical Position/1 -> Theta/1
  Speed Measurement/1 -> IIR Filter/1
  Pos_Sim/1 -> Mechanical to Electrical Position/1, Speed Measurement/1
  IIR Filter/1 -> Speed/1

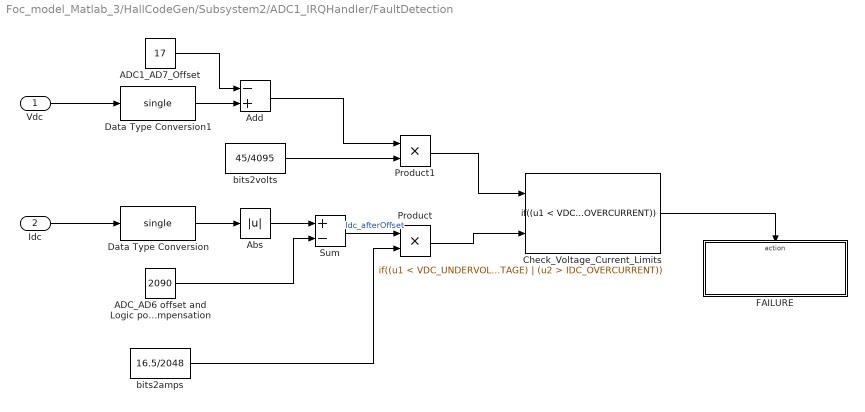
== system Foc_model_Matlab_3/HallCodeGen/Subsystem2/ADC1_IRQHandler/FaultDetection ==
  Vdc : Inport
  Idc : Inport  Port=2
  ADC1_AD7_Offset : Constant  Value=17  OutDataTypeStr=single
  ADC_AD6 offset and Logic power supply compensation : Constant  Value=2090  OutDataTypeStr=single
  Abs : Abs  SaturateOnIntegerOverflow=off
  Add : Sum  Inputs=-+  OutMin=0  OutMax=4095  OutDataTypeStr=single  AccumDataTypeStr=single  InputSameDT=on
  Check_Voltage_Current_Limits : If  NumInputs=2  IfExpression=(u1 < VDC_UNDERVOLTAGE) | (u1 > VDC_OVERVOLTAGE) | (u2 > IDC_OVERCURRENT)  ShowElse=off
  Data Type Conversion : DataTypeConversion  OutDataTypeStr=single  SaturateOnIntegerOverflow=off  RndMeth=Floor
  Data Type Conversion1 : DataTypeConversion  OutDataTypeStr=single  SaturateOnIntegerOverflow=off  RndMeth=Floor
  FAILURE : Subsystem  TreatAsAtomicUnit=on
  Product : Product  OutDataTypeStr=single
  Product1 : Product  OutDataTypeStr=single
  Sum : Sum  Inputs=+-  OutDataTypeStr=single  AccumDataTypeStr=single
  bits2amps : Constant  Value=16.5/2048  OutDataTypeStr=single
  bits2volts : Constant  Value=45/4095  OutDataTypeStr=single
  wires:
  Check_Voltage_Current_Limits/1 -> FAILURE/Action
  Idc/1 -> Data Type Conversion/1
  Data Type Conversion/1 -> Abs/1
  Vdc/1 -> Data Type Conversion1/1
  Abs/1 -> Sum/1
  ADC_AD6 offset and Logic power supply compensation/1 -> Sum/2
  Sum/1 -> Product/1  "Idc_afterOffset"
  Product/1 -> Check_Voltage_Current_Limits/2
  bits2amps/1 -> Product/2
  ADC1_AD7_Offset/1 -> Add/1
  Data Type Conversion1/1 -> Add/2
  bits2volts/1 -> Product1/2
  Add/1 -> Product1/1
  Product1/1 -> Check_Voltage_Current_Limits/1
